simulink model "SISO_slx"  (R2024a)
settings: Solver=VariableStepAuto  StartTime=0.0  StopTime=t_sim  RelTol=1e-3
values from neighbouring files (symbols this model uses):
  C = [0 1 1]    [SISO.m]    (also in invertedPendulum.m = [-1 0 0 0; invertedPendulumSys.m = [-1 0 0 0)
  k_q = K(1)    [SISO.m]
  k_x = K(2:end)    [SISO.m]
libraries: cstblocks x1
settings Model: Creator=jiaxingzhang  LastModifiedBy=lorenzo
settings ModelReferenceCC: EnableRefExpFcnMdlSchedulingChecks=on
settings RTWCC: GPUComputeCapability=3.5

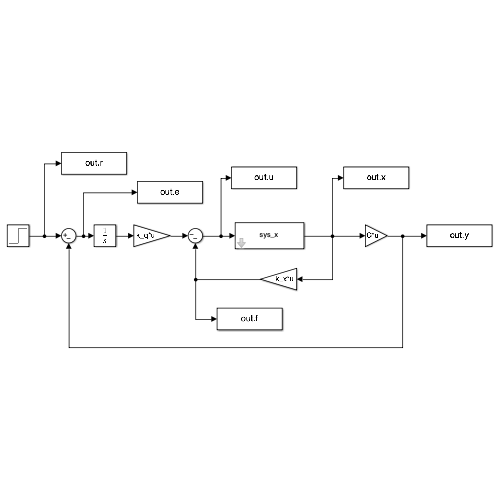
[thumbnail: Simulink's stored preview of the top-level diagram]
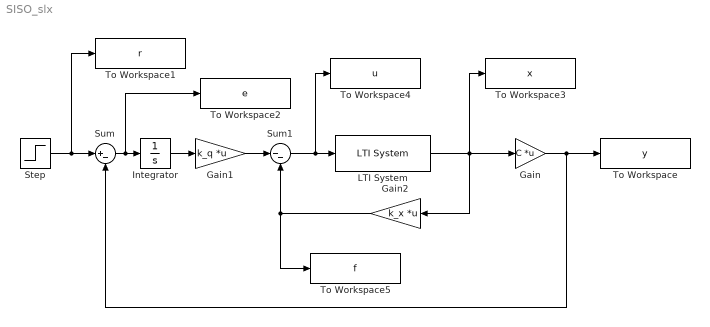
== system SISO_slx ==
  Gain : Gain  Gain=C  Multiplication=Matrix(K*u)
  Gain1 : Gain  Gain=k_q  Multiplication=Matrix(K*u)
  Gain2 : Gain  Gain=k_x  Multiplication=Matrix(K*u)
  Integrator : Integrator
  LTI System : cstblocks/LTI System  sys=sys_x  IC=[]  PadeOrder=0
  Step : Step  Before=1  SampleTime=0
  Sum : Sum  Inputs=|+-
  Sum1 : Sum  Inputs=|--
  To Workspace : ToWorkspace  VariableName=y  SaveFormat=Timeseries  SampleTime=-1
  To Workspace1 : ToWorkspace  VariableName=r  SaveFormat=Timeseries  SampleTime=-1
  To Workspace2 : ToWorkspace  VariableName=e  SaveFormat=Timeseries  SampleTime=-1
  To Workspace3 : ToWorkspace  VariableName=x  SaveFormat=Timeseries  SampleTime=-1
  To Workspace4 : ToWorkspace  VariableName=u  SaveFormat=Timeseries  SampleTime=-1
  To Workspace5 : ToWorkspace  VariableName=f  SaveFormat=Timeseries  SampleTime=-1
  wires:
  LTI System/1 -> To Workspace3/1, Gain/1, Gain2/1
  Gain/1 -> Sum/2, To Workspace/1
  Integrator/1 -> Gain1/1
  Sum/1 -> To Workspace2/1, Integrator/1
  Step/1 -> To Workspace1/1, Sum/1
  Gain1/1 -> Sum1/1
  Sum1/1 -> To Workspace4/1, LTI System/1
  Gain2/1 -> To Workspace5/1, Sum1/2
